simulink model "A18_SEPIC_converter"  (R2017a)
settings: Solver=ode4  StartTime=0.0  StopTime=0.15  FixedStep=1e-8  RelTol=1e-3  EnableMultiTasking=on
InitFcn:
  | V=10
  | L1=0.325e-3
  | L2=0.325e-3
  | C1=0.0726e-3
  | C2=0.102e-3
  | R=12
  | Pe=1/25000
  | w=61
libraries: powerlib x15
settings Model: Creator=s18elme04  LastModifiedBy=A_M
settings DataIOCC: LimitDataPoints=on  SaveFormat=Array
settings OptimizationCC: ExpressionDepthLimit=2147483647  InitFltsAndDblsToZero=on  LifeSpan=inf
settings DebuggingCC: UnderspecifiedInitializationDetection=Classic  MergeDetectMultiDrivingBlocksExec=none  SolverPrmCheckMsg=warning  FcnCallInpInsideContextMsg=warning  StateNameClashWarn=warning  SFUnexpectedBacktrackingDiag=warning  SFNoUnconditionalDefaultTransitionDiag=warning  SFExecutionAtInitializationDiag=none
settings HardwareCC: ProdBitPerPointer=32  ProdBitPerSizeT=32  ProdBitPerPtrDiffT=32  ProdLargestAtomicFloat=None  ProdIntDivRoundTo=Undefined  ProdEndianess=Unspecified  ProdWordSize=32  ProdHWDeviceType=32-bit Generic
settings ModelReferenceCC: PropagateSignalLabelsOutOfModel=off
settings GRTTargetCC: TargetLangStandard=C89/C90 (ANSI)  CombineOutputUpdateFcns=off  GRTInterface=on
settings ConfigComp: CovMetricSettings=dw  CovHtmlReporting=on  CovSaveCumulativeToWorkspaceVar=on  CovSaveSingleToWorkspaceVar=on  CovExternalEMLEnable=off

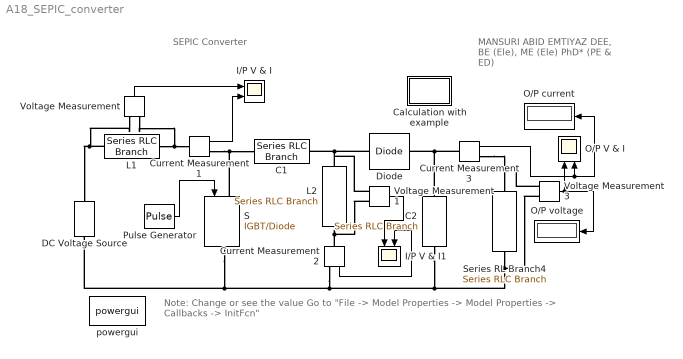
== system A18_SEPIC_converter ==
  note: Note: Change or see the value
      | Go to "File -> Model Properties -> Model Properties -> Callbacks -> InitFcn"
  note: SEPIC Converter
  note: MANSURI ABID EMTIYAZ
      | DEE, BE (Ele), ME (Ele)
      | PhD* (PE & ED)
  C1 : powerlib/Elements/Series RLC Branch  LConnTagsString=__new0  RConnTagsString=__new0  BranchType=C  Resistance=1  Inductance=1e-3  SetiL0=off  InitialCurrent=0  Capacitance=C1  Setx0=off  InitialVoltage=0  Measurements=None
  C2 : powerlib/Elements/Series RLC Branch  LConnTagsString=__new0  RConnTagsString=__new0  BranchType=C  Resistance=1  Inductance=1e-3  SetiL0=off  InitialCurrent=0  Capacitance=C2  Setx0=off  InitialVoltage=0  Measurements=None
  Calculation with example : Subsystem
  Current Measurement1 : powerlib/Measurements/Current Measurement  PhasorSimulation=off  OutputType=Complex  PSBequivalent=0
  Current Measurement2 : powerlib/Measurements/Current Measurement  PhasorSimulation=off  OutputType=Complex  PSBequivalent=0
  Current Measurement3 : powerlib/Measurements/Current Measurement  PhasorSimulation=off  OutputType=Complex  PSBequivalent=0
  DC Voltage Source : powerlib/Electrical Sources/DC Voltage Source  Amplitude=V  Measurements=None
  Diode : powerlib/Power Electronics/Diode  Ron=0.001  Lon=0  Vf=0.1  IC=0  UseSnubber=off  Rs=500  Cs=250e-9  Measurements=off
  I/P V & I : Scope  NumInputPorts=2
  I/P V & I1 : Scope  NumInputPorts=2
  L1 : powerlib/Elements/Series RLC Branch  LConnTagsString=__new0  RConnTagsString=__new0  BranchType=L  Resistance=1  Inductance=L1  SetiL0=off  InitialCurrent=0  Capacitance=1e-6  Setx0=off  InitialVoltage=0  Measurements=None
  L2 : powerlib/Elements/Series RLC Branch  LConnTagsString=__new0  RConnTagsString=__new0  BranchType=L  Resistance=1  Inductance=L2  SetiL0=off  InitialCurrent=0  Capacitance=1e-6  Setx0=off  InitialVoltage=0  Measurements=None
  O/P V & I : Scope  NumInputPorts=2
  O/P current : Display
  O/P voltage : Display
  Pulse Generator : DiscretePulseGenerator  PulseType=Time based  Period=Pe  PulseWidth=w
  S : powerlib/Power Electronics/IGBT//Diode  Ron=1e-3  Rs=1e5  Cs=inf  Measurements=off
  Series RL Branch4 : powerlib/Elements/Series RLC Branch  LConnTagsString=__new0  RConnTagsString=__new0  BranchType=R  Resistance=R  Inductance=1e-3  SetiL0=off  InitialCurrent=0  Capacitance=1e-6  Setx0=off  InitialVoltage=0  Measurements=None
  Voltage Measurement : powerlib/Measurements/Voltage Measurement  PhasorSimulation=off  OutputType=Complex  PSBequivalent=0
  Voltage Measurement1 : powerlib/Measurements/Voltage Measurement  PhasorSimulation=off  OutputType=Complex  PSBequivalent=0
  Voltage Measurement3 : powerlib/Measurements/Voltage Measurement  PhasorSimulation=off  OutputType=Complex  PSBequivalent=0
  powergui : powerlib/powergui  Priority=1  SimulationMode=Discrete  SampleTime=1e-8  frequency=60  Iterations=50  frequencyindice=0  Pbase=100e6  ErrMax=1e-4  UnitsV=kV  UnitsW=MW  buscounter=0  FunctionMessages=off  echomessages=off  EnableUseOfTLC=off  CurrentSourceSwitches=off  DisableSnubberDevices=off  DisableRonSwitches=off  DisableVfSwitches=off  DisplayEquations=off  SolverType=Tustin/Backward Euler (TBE)  Interpol=off  ExternalGateDelay=off  methode=off  Ts=100  x0status=blocks  SPID=on  SwTol=0  HookPort=off  RestoreLinks=warning  ResistiveCurrentMeasurement=off  Frange=[0:2:500]  Ylog=off  Xlog=on  ShowGrid=off  save=off  variable=ZData  structure=0  ZoomFFT=off  StartTime=0.0  cycles=1  DisplayStyle=1  fundamental=60  FreqAxis=off  MaxFrequency=1000  frequencyindicesteady=1  RmsSteady=1  display=off
  wires:
  Voltage Measurement/1 -> I/P V & I/1
  Current Measurement1/1 -> I/P V & I/2
  Pulse Generator/1 -> S/1
  Voltage Measurement3/1 -> O/P voltage/1, O/P V & I/1
  Voltage Measurement1/1 -> I/P V & I1/1
  Current Measurement2/1 -> I/P V & I1/2
  Current Measurement3/1 -> O/P V & I/2, O/P current/1
  connections:
  Current Measurement2/LConn1 -- L2/RConn1 -- Voltage Measurement1/LConn2
  L1/LConn1 -- DC Voltage Source/RConn1 -- Voltage Measurement/LConn1
  L1/RConn1 -- Voltage Measurement/LConn2 -- Current Measurement1/LConn1
  Current Measurement1/RConn1 -- C1/LConn1 -- S/LConn1
  Diode/LConn1 -- Voltage Measurement1/LConn1 -- L2/LConn1 -- C1/RConn1
  Current Measurement3/LConn1 -- C2/LConn1 -- Diode/RConn1
  Current Measurement3/RConn1 -- Voltage Measurement3/LConn1 -- Series RL Branch4/LConn1
  Series RL Branch4/RConn1 -- Voltage Measurement3/LConn2 -- C2/RConn1 -- Current Measurement2/RConn1 -- S/RConn1 -- DC Voltage Source/LConn1

== system A18_SEPIC_converter/Calculation with example ==
  note: Equations and it's solution for Calculation of R L and C is explain in below link
      | " https://www.researchgate.net/publication/342865821_Basic_SEPIC_Converter_Calculation_of_R_L_and_C_-_Hand_outs "
